simulink model "bh_road_in_simulink"  (R2021a)
settings: Solver=VariableStepAuto  StartTime=0.0  StopTime=70  RelTol=1e-3
settings Model: Creator=bhorton  LastModifiedBy=bhorton

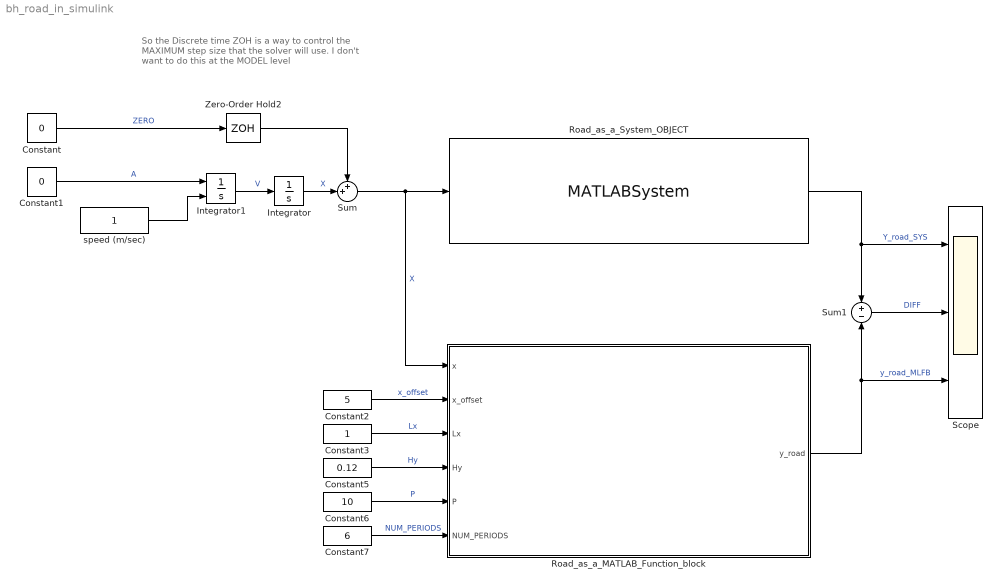
== system bh_road_in_simulink ==
  note: So the Discrete time ZOH is a way to control
      | the MAXIMUM step size that the solver will use.
      |
      | I don't want to do this at the MODEL level
  Constant : Constant  Value=0
  Constant1 : Constant  Value=0
  Constant2 : Constant  Value=5
  Constant3 : Constant
  Constant5 : Constant  Value=0.12
  Constant6 : Constant  Value=10
  Constant7 : Constant  Value=6
  Integrator : Integrator
  Integrator1 : Integrator  InitialConditionSource=external
  Road_as_a_MATLAB_Function_block : MATLAB Function  TreatAsAtomicUnit=on
  Road_as_a_System_OBJECT : MATLABSystem  System=bh_road_hump_A_SYSO  Hy=0.12  Lx=1  P=10  x_offset=5  NUM_PERIODS=6  SimulateUsing=Interpreted execution
      settings: AttributesFormatString=|
      | x_offset = %<x_offset> (m)
      | L_x = %<Lx> (m)
      | H_y = %<Hy> (m)
      | P =%<P> (m)
      | NUM_PERIODS = %<NUM_PERIODS>
      mask Type: bh_road_hump_A_SYSO
      mask Display:
      | disp('bh_road_hump_A_SYSO');
      | port_label('input',1,'X_car');
      | port_label('output',1,'Y_road');
  Scope : Scope  NumInputPorts=3
  Sum : Sum  Inputs=++|
  Sum1 : Sum  Inputs=+|-
  Zero-Order Hold2 : ZeroOrderHold  SampleTime=1/1000
      settings: AttributesFormatString=dT =%<SampleTime>
  speed (m/sec) : Constant
  wires:
  Zero-Order Hold2/1 -> Sum/1
  Constant/1 -> Zero-Order Hold2/1  "ZERO"
  Constant1/1 -> Integrator1/1  "A"
  speed (m/sec)/1 -> Integrator1/2
  Integrator1/1 -> Integrator/1  "V"
  Road_as_a_System_OBJECT/1 -> Sum1/1, Scope/1  "Y_road_SYS"
  Integrator/1 -> Sum/2  "X"
  Sum/1 -> Road_as_a_MATLAB_Function_block/1(x), Road_as_a_System_OBJECT/1  "X"
  Constant2/1 -> Road_as_a_MATLAB_Function_block/2(x_offset)  "x_offset"
  Constant3/1 -> Road_as_a_MATLAB_Function_block/3(Lx)  "Lx"
  Constant6/1 -> Road_as_a_MATLAB_Function_block/5(P)  "P"
  Constant5/1 -> Road_as_a_MATLAB_Function_block/4(Hy)  "Hy"
  Road_as_a_MATLAB_Function_block/1(y_road) -> Scope/3, Sum1/2  "y_road_MLFB"
  Sum1/1 -> Scope/2  "DIFF"
  Constant7/1 -> Road_as_a_MATLAB_Function_block/6(NUM_PERIODS)  "NUM_PERIODS"

== matlab function bh_road_in_simulink/Road_as_a_MATLAB_Function_block ==
  data: x input; y_road output; x_offset input; Lx input; Hy input; P input; NUM_PERIODS input
function y_road = fcn(x, x_offset, Lx, Hy, P, NUM_PERIODS)
 
   y_road            = LOC_road_half_sine(x, x_offset, Lx, Hy, P);
   
   tf_x_beyond_block = x > (x_offset + P*NUM_PERIODS);
            
   y_road(tf_x_beyond_block) = 0;
end
%==========================================================================
% SUBFUNCTIONS
%==========================================================================
function y = LOC_road_half_sine(x, x_offset, Lx, Hy, P)
  
   Xc = x - x_offset;
   
   y  = zeros(size(Xc));
   N  = length(Xc);
   
   for kk=1:N

       x_pnt = Xc(kk);

      if(x_pnt<0)
           y(kk) = 0;
      else % x > 0
           x_mod = mod(x_pnt,P); 
           
          if(x_mod <= Lx & x_mod>=0)
              
              y(kk) = Hy * sin(pi*x_mod/Lx);
              
          elseif(x_mod > Lx & x_mod <= P) 
              y(kk) = 0;
          end
      end
   end % for
   
end % function
%==========================================================================
